simulink model "Buck_DCM_z"  (R2020a)
settings: Solver=FixedStepAuto  StartTime=0.0  StopTime=20  FixedStep=T  RelTol=1e-3
undefined symbols (not defined in the file): C, Iumax, J, Ki_I, Ki_IL, Kp_I, Kp_IL, Kp_Uc, Kp_W, Kphi, L, Lu, rL, Ru, T, Ubat
libraries: powerlib_meascontrol x3
settings Model: Creator=Nguyen Tung  LastModifiedBy=Nguyen Tung

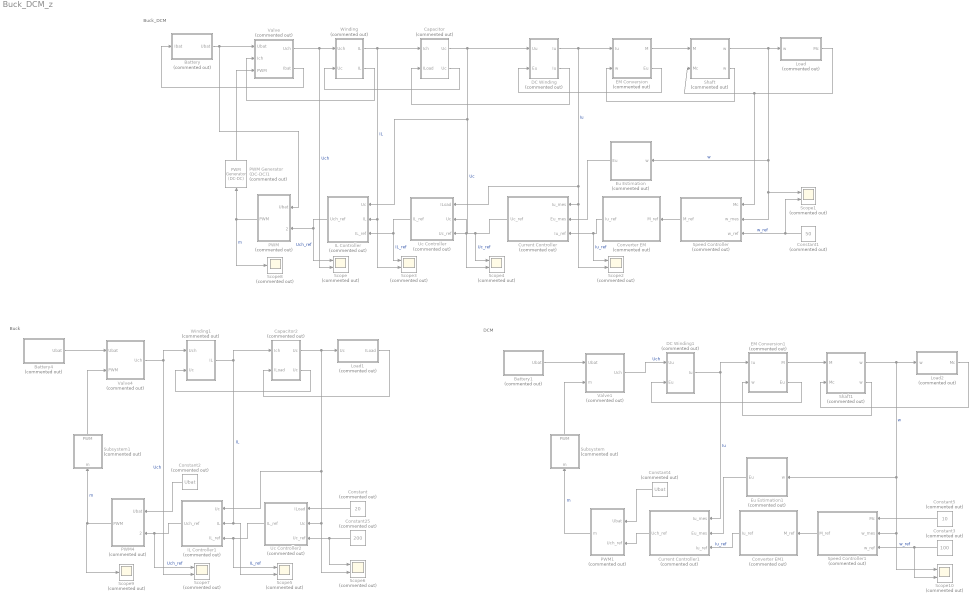
== system Buck_DCM_z ==
  note: DCM
  note: Buck
  note: Buck_DCM
  Battery : Subsystem  Commented=on  AncestorBlock=simulink/REM/SE
      mask Display:
      | plot(0,0,100,100, 1.2*[50,57.68,60.77,63.08,64.97,66.58,68,69.26,70.4, 	71.42,72.36,78.28,80,78.28,72.36,71.42,70.4, 	69.26,68,66.58,64.97,63.08,60.77,57.68,50,42.32, 	39.23,36.92,35.03,33.42,32,30.74,29.6,28.58, 	27.64,21.72,20,21.72,27.64,28.58,29.6,30.74,32, 	33.42,35.03,36.92,39.23,42.32,50]-10, 1.2*[20,21,22,23,24,25,26,27,28,29,30,40,50,60,70,71,72, 	73,74,75,76,77,78,79,80,79,78,77,76,75,74,73,72, 	71,70,60,50,40,30,29,28,27,26,25,24,23,22,21,20]-10)
      | disp('ES')
  Battery1 : Subsystem  Commented=on  AncestorBlock=simulink/REM/SE
      mask Display:
      | plot(0,0,100,100, 1.2*[50,57.68,60.77,63.08,64.97,66.58,68,69.26,70.4, 	71.42,72.36,78.28,80,78.28,72.36,71.42,70.4, 	69.26,68,66.58,64.97,63.08,60.77,57.68,50,42.32, 	39.23,36.92,35.03,33.42,32,30.74,29.6,28.58, 	27.64,21.72,20,21.72,27.64,28.58,29.6,30.74,32, 	33.42,35.03,36.92,39.23,42.32,50]-10, 1.2*[20,21,22,23,24,25,26,27,28,29,30,40,50,60,70,71,72, 	73,74,75,76,77,78,79,80,79,78,77,76,75,74,73,72, 	71,70,60,50,40,30,29,28,27,26,25,24,23,22,21,20]-10)
      | disp('ES')
  Battery4 : Subsystem  Commented=on  AncestorBlock=simulink/REM/SE
      mask Display:
      | plot(0,0,100,100, 1.2*[50,57.68,60.77,63.08,64.97,66.58,68,69.26,70.4, 	71.42,72.36,78.28,80,78.28,72.36,71.42,70.4, 	69.26,68,66.58,64.97,63.08,60.77,57.68,50,42.32, 	39.23,36.92,35.03,33.42,32,30.74,29.6,28.58, 	27.64,21.72,20,21.72,27.64,28.58,29.6,30.74,32, 	33.42,35.03,36.92,39.23,42.32,50]-10, 1.2*[20,21,22,23,24,25,26,27,28,29,30,40,50,60,70,71,72, 	73,74,75,76,77,78,79,80,79,78,77,76,75,74,73,72, 	71,70,60,50,40,30,29,28,27,26,25,24,23,22,21,20]-10)
      | disp('ES')
  Capacitor : Subsystem  Commented=on  AncestorBlock=simulink/REM/EA  mask(CM){}
      mask Display: plot(0,0,100,100,[10,10,90,90,10],[90,10,10,90,90], [10,90],[10,90])
  Capacitor2 : Subsystem  Commented=on  AncestorBlock=simulink/REM/EA  mask(CM){}
      mask Display: plot(0,0,100,100,[10,10,90,90,10],[90,10,10,90,90], [10,90],[10,90])
  Constant : Constant  Commented=on  Value=20
  Constant1 : Constant  Commented=on  Value=50
  Constant2 : Constant  Commented=on  Value=Ubat
  Constant25 : Constant  Commented=on  Value=200  SampleTime=T
  Constant3 : Constant  Commented=on  Value=100
  Constant4 : Constant  Commented=on  Value=Ubat
  Constant5 : Constant  Commented=on  Value=10
  Converter EM : Subsystem  Commented=on  AncestorBlock=simulink/SMC/Inversion EC avec mesure
      mask Display: plot(0,0,100,100,[10,30,90,70,10],[90,10,10,90,90])
  Converter EM1 : Subsystem  Commented=on  AncestorBlock=simulink/SMC/Inversion EC avec mesure
      mask Display: plot(0,0,100,100,[10,30,90,70,10],[90,10,10,90,90])
  Current Controller : Subsystem  Commented=on  AncestorBlock=simulink/SMC/Asservissement Correcteur IP
      mask Display: plot(0,0,100,100, [10,30,90,70,10,90],[90,10,10,90,90,10])
  Current Controller1 : Subsystem  Commented=on  AncestorBlock=simulink/SMC/Asservissement Correcteur IP
      mask Display: plot(0,0,100,100, [10,30,90,70,10,90],[90,10,10,90,90,10])
  DC Winding : Subsystem  Commented=on  AncestorBlock=simulink/REM/EA  mask(CM){}
      mask Display: plot(0,0,100,100,[10,10,90,90,10],[90,10,10,90,90], [10,90],[10,90])
  DC Winding1 : Subsystem  Commented=on  AncestorBlock=simulink/REM/EA  mask(CM){}
      mask Display: plot(0,0,100,100,[10,10,90,90,10],[90,10,10,90,90], [10,90],[10,90])
  EM Conversion : Subsystem  Commented=on  AncestorBlock=simulink/REM/EC EM
      mask Display: plot(0,0,100,100, 1.4*[50,57.68,60.77,63.08,64.97,66.58,68,69.26,70.4, 	71.42,72.36,78.28,80,78.28,72.36,71.42,70.4, 	69.26,68,66.58,64.97,63.08,60.77,57.68,50,42.32, 	39.23,36.92,35.03,33.42,32,30.74,29.6,28.58, 	27.64,21.72,20,21.72,27.64,28.58,29.6,30.74,32, 	33.42,35.03,36.92,39.23,42.32,50]-20, 1.4*[20,21,22,23,24,25,26,27,28,29,30,40,50,60,70,71,72, 	73,74,75,76,77,78,79,80,79,78,77,76,75,74,73,72, 	71,70,60,50,40,30,29,28,27,26,25,24,23,22,21,20]-20)
  EM Conversion1 : Subsystem  Commented=on  AncestorBlock=simulink/REM/EC EM
      mask Display: plot(0,0,100,100, 1.4*[50,57.68,60.77,63.08,64.97,66.58,68,69.26,70.4, 	71.42,72.36,78.28,80,78.28,72.36,71.42,70.4, 	69.26,68,66.58,64.97,63.08,60.77,57.68,50,42.32, 	39.23,36.92,35.03,33.42,32,30.74,29.6,28.58, 	27.64,21.72,20,21.72,27.64,28.58,29.6,30.74,32, 	33.42,35.03,36.92,39.23,42.32,50]-20, 1.4*[20,21,22,23,24,25,26,27,28,29,30,40,50,60,70,71,72, 	73,74,75,76,77,78,79,80,79,78,77,76,75,74,73,72, 	71,70,60,50,40,30,29,28,27,26,25,24,23,22,21,20]-20)
  Eu Estimation : Subsystem  Commented=on  AncestorBlock=simulink/REM/EC EM
      mask Display: plot(0,0,100,100, 1.4*[50,57.68,60.77,63.08,64.97,66.58,68,69.26,70.4, 	71.42,72.36,78.28,80,78.28,72.36,71.42,70.4, 	69.26,68,66.58,64.97,63.08,60.77,57.68,50,42.32, 	39.23,36.92,35.03,33.42,32,30.74,29.6,28.58, 	27.64,21.72,20,21.72,27.64,28.58,29.6,30.74,32, 	33.42,35.03,36.92,39.23,42.32,50]-20, 1.4*[20,21,22,23,24,25,26,27,28,29,30,40,50,60,70,71,72, 	73,74,75,76,77,78,79,80,79,78,77,76,75,74,73,72, 	71,70,60,50,40,30,29,28,27,26,25,24,23,22,21,20]-20)
  Eu Estimation1 : Subsystem  Commented=on  AncestorBlock=simulink/REM/EC EM
      mask Display: plot(0,0,100,100, 1.4*[50,57.68,60.77,63.08,64.97,66.58,68,69.26,70.4, 	71.42,72.36,78.28,80,78.28,72.36,71.42,70.4, 	69.26,68,66.58,64.97,63.08,60.77,57.68,50,42.32, 	39.23,36.92,35.03,33.42,32,30.74,29.6,28.58, 	27.64,21.72,20,21.72,27.64,28.58,29.6,30.74,32, 	33.42,35.03,36.92,39.23,42.32,50]-20, 1.4*[20,21,22,23,24,25,26,27,28,29,30,40,50,60,70,71,72, 	73,74,75,76,77,78,79,80,79,78,77,76,75,74,73,72, 	71,70,60,50,40,30,29,28,27,26,25,24,23,22,21,20]-20)
  IL Controller : Subsystem  Commented=on  AncestorBlock=simulink/SMC/Asservissement Correcteur IP
      mask Display: plot(0,0,100,100, [10,30,90,70,10,90],[90,10,10,90,90,10])
  IL Controller1 : Subsystem  Commented=on  AncestorBlock=simulink/SMC/Asservissement Correcteur IP
      mask Display: plot(0,0,100,100, [10,30,90,70,10,90],[90,10,10,90,90,10])
  Load : Subsystem  Commented=on  AncestorBlock=simulink/REM/SE
      mask Display:
      | plot(0,0,100,100, 1.2*[50,57.68,60.77,63.08,64.97,66.58,68,69.26,70.4, 	71.42,72.36,78.28,80,78.28,72.36,71.42,70.4, 	69.26,68,66.58,64.97,63.08,60.77,57.68,50,42.32, 	39.23,36.92,35.03,33.42,32,30.74,29.6,28.58, 	27.64,21.72,20,21.72,27.64,28.58,29.6,30.74,32, 	33.42,35.03,36.92,39.23,42.32,50]-10, 1.2*[20,21,22,23,24,25,26,27,28,29,30,40,50,60,70,71,72, 	73,74,75,76,77,78,79,80,79,78,77,76,75,74,73,72, 	71,70,60,50,40,30,29,28,27,26,25,24,23,22,21,20]-10)
      | disp('MS')
  Load1 : Subsystem  Commented=on  AncestorBlock=simulink/REM/SE
      mask Display:
      | plot(0,0,100,100, 1.2*[50,57.68,60.77,63.08,64.97,66.58,68,69.26,70.4, 	71.42,72.36,78.28,80,78.28,72.36,71.42,70.4, 	69.26,68,66.58,64.97,63.08,60.77,57.68,50,42.32, 	39.23,36.92,35.03,33.42,32,30.74,29.6,28.58, 	27.64,21.72,20,21.72,27.64,28.58,29.6,30.74,32, 	33.42,35.03,36.92,39.23,42.32,50]-10, 1.2*[20,21,22,23,24,25,26,27,28,29,30,40,50,60,70,71,72, 	73,74,75,76,77,78,79,80,79,78,77,76,75,74,73,72, 	71,70,60,50,40,30,29,28,27,26,25,24,23,22,21,20]-10)
      | disp('MS')
  Load2 : Subsystem  Commented=on  AncestorBlock=simulink/REM/SE
      mask Display:
      | plot(0,0,100,100, 1.2*[50,57.68,60.77,63.08,64.97,66.58,68,69.26,70.4, 	71.42,72.36,78.28,80,78.28,72.36,71.42,70.4, 	69.26,68,66.58,64.97,63.08,60.77,57.68,50,42.32, 	39.23,36.92,35.03,33.42,32,30.74,29.6,28.58, 	27.64,21.72,20,21.72,27.64,28.58,29.6,30.74,32, 	33.42,35.03,36.92,39.23,42.32,50]-10, 1.2*[20,21,22,23,24,25,26,27,28,29,30,40,50,60,70,71,72, 	73,74,75,76,77,78,79,80,79,78,77,76,75,74,73,72, 	71,70,60,50,40,30,29,28,27,26,25,24,23,22,21,20]-10)
      | disp('MS')
  PWM : Subsystem  Commented=on  AncestorBlock=simulink/SMC/Inversion EC avec mesure
      mask Display: plot(0,0,100,100,[10,30,90,70,10],[90,10,10,90,90])
  PWM Generator (DC-DC)1 : powerlib_meascontrol/Pulse & Signal Generators/PWM Generator (DC-DC)  Commented=on  Fsw=1000  Ts=T
  PWM1 : Subsystem  Commented=on  AncestorBlock=simulink/SMC/Inversion EC avec mesure
      mask Display: plot(0,0,100,100,[10,30,90,70,10],[90,10,10,90,90])
  PWM4 : Subsystem  Commented=on  AncestorBlock=simulink/SMC/Inversion EC avec mesure
      mask Display: plot(0,0,100,100,[10,30,90,70,10],[90,10,10,90,90])
  Scope{,1..7,10} (9 alike) : Scope  Commented=on  NumInputPorts=2
  Scope8 : Scope  Commented=on
  Scope9 : Scope  Commented=on
  Shaft : Subsystem  Commented=on  AncestorBlock=simulink/REM/EA  mask(CM){}
      mask Display: plot(0,0,100,100,[10,10,90,90,10],[90,10,10,90,90], [10,90],[10,90])
  Shaft1 : Subsystem  Commented=on  AncestorBlock=simulink/REM/EA  mask(CM){}
      mask Display: plot(0,0,100,100,[10,10,90,90,10],[90,10,10,90,90], [10,90],[10,90])
  Speed Controller : Subsystem  Commented=on  AncestorBlock=simulink/SMC/Asservissement Correcteur IP
      mask Display: plot(0,0,100,100, [10,30,90,70,10,90],[90,10,10,90,90,10])
  Speed Controller1 : Subsystem  Commented=on  AncestorBlock=simulink/SMC/Asservissement Correcteur IP
      mask Display: plot(0,0,100,100, [10,30,90,70,10,90],[90,10,10,90,90,10])
  Subsystem : Subsystem  Commented=on
  Subsystem1 : Subsystem  Commented=on
  Uc Controller : Subsystem  Commented=on  AncestorBlock=simulink/SMC/Asservissement Correcteur IP
      mask Display: plot(0,0,100,100, [10,30,90,70,10,90],[90,10,10,90,90,10])
  Uc Controller2 : Subsystem  Commented=on  AncestorBlock=simulink/SMC/Asservissement Correcteur IP
      mask Display: plot(0,0,100,100, [10,30,90,70,10,90],[90,10,10,90,90,10])
  Valve : Subsystem  Commented=on  AncestorBlock=simulink/REM/EC Elec  mask(Hacheur){}
      mask Display: plot(0,0,100,100,[10,10,90,90,10],[90,10,10,90,90])
  Valve1 : Subsystem  Commented=on  AncestorBlock=simulink/REM/EC Elec  mask(Hacheur){}
      mask Display: plot(0,0,100,100,[10,10,90,90,10],[90,10,10,90,90])
  Valve4 : Subsystem  Commented=on  AncestorBlock=simulink/REM/EC Elec  mask(Hacheur){}
      mask Display: plot(0,0,100,100,[10,10,90,90,10],[90,10,10,90,90])
  Winding : Subsystem  Commented=on  AncestorBlock=simulink/REM/EA  mask(CM){}
      mask Display: plot(0,0,100,100,[10,10,90,90,10],[90,10,10,90,90], [10,90],[10,90])
  Winding1 : Subsystem  Commented=on  AncestorBlock=simulink/REM/EA  mask(CM){}
      mask Display: plot(0,0,100,100,[10,10,90,90,10],[90,10,10,90,90], [10,90],[10,90])
  wires:
  Capacitor/1(Uc) -> DC Winding/1(Uu), IL Controller/1(Uc), Scope4/2, Uc Controller/2(Uc)  "Uc"
  Shaft/1(w) -> Load/1(w), Speed Controller/2(w_mes), Scope1/1, Eu Estimation/1(w)  "w"
  Winding/1(IL) -> Capacitor/1(Ich), Scope3/2, IL Controller/2(IL)  "IL"
  Valve/1(Uch) -> Scope/2, Winding/1(Uch)  "Uch"
  Speed Controller/1(M_ref) -> Converter EM/1(M_ref)
  PWM/1(PWM) -> Scope8/1, PWM Generator (DC-DC)1/1  "m"
  Valve/2(Ibat) -> Battery/1(Ibat)
  Load/1(Mc) -> Speed Controller/1(Mc), Shaft/2(Mc)
  Converter EM/1(Iu_ref) -> Current Controller/3(Iu_ref), Scope2/1  "Iu_ref"
  Uc Controller/1(IL_ref) -> Scope3/1, IL Controller/3(IL_ref)  "IL_ref"
  Shaft/2("w ") -> EM Conversion/2(w)
  EM Conversion/1(M) -> Shaft/1(M)
  EM Conversion/2(Eu) -> DC Winding/2(Eu)
  IL Controller/1(Uch_ref) -> Scope/1, PWM/2(Uch_ref)  "Uch_ref"
  DC Winding/2("Iu ") -> Capacitor/2(ILoad)
  Eu Estimation/1(Eu) -> Current Controller/2(Eu_mes)
  Constant1/1 -> Speed Controller/3(w_ref), Scope1/2  "w_ref"
  DC Winding/1(Iu) -> EM Conversion/1(Iu), Scope2/2, Current Controller/1(Iu_mes), Uc Controller/1(ILoad)  "Iu"
  Battery/1(Ubat) -> Valve/1(Ubat), PWM/1(Ubat)
  Winding/2("IL ") -> Valve/2(Ich)
  Capacitor/2("Uc ") -> Winding/2(Uc)
  Current Controller/1(Uc_ref) -> Scope4/1, Uc Controller/3(Uc_ref)  "Uc_ref"
  PWM4/1(PWM) -> Scope9/1, Subsystem1/1(m)  "m"
  Load1/1(ILoad) -> Capacitor2/2(ILoad)
  Battery4/1(Ubat) -> Valve4/1(Ubat)
  Capacitor2/1(Uc) -> Load1/1(Uc), IL Controller1/1(Uc), Scope6/2, Uc Controller2/2(Uc)
  Winding1/1(IL) -> Capacitor2/1(Ich), Scope5/2, IL Controller1/2(IL)  "IL"
  Valve4/1(Uch) -> Winding1/1(Uch), Scope7/2  "Uch"
  IL Controller1/1(Uch_ref) -> Scope7/1, PWM4/2(Uch_ref)  "Uch_ref"
  Uc Controller2/1(IL_ref) -> Scope5/1, IL Controller1/3(IL_ref)  "IL_ref"
  Capacitor2/2("Uc ") -> Winding1/2(Uc)
  Constant25/1 -> Scope6/1, Uc Controller2/3(Uc_ref)
  PWM Generator (DC-DC)1/1 -> Valve/3(PWM)
  Constant/1 -> Uc Controller2/1(ILoad)
  Constant2/1 -> PWM4/1(Ubat)
  Converter EM1/1(Iu_ref) -> Current Controller1/3(Iu_ref)  "Iu_ref"
  Shaft1/1(w) -> Load2/1(w), Scope10/1, Speed Controller1/2(w_mes), Eu Estimation1/1(w)  "w"
  DC Winding1/1(Iu) -> EM Conversion1/1(Iu), Current Controller1/1(Iu_mes)  "Iu"
  EM Conversion1/2(Eu) -> DC Winding1/2(Eu)
  Eu Estimation1/1(Eu) -> Current Controller1/2(Eu_mes)
  Constant3/1 -> Speed Controller1/3(w_ref), Scope10/2  "w_ref"
  EM Conversion1/1(M) -> Shaft1/1(M)
  Shaft1/2("w ") -> EM Conversion1/2(w)
  Speed Controller1/1(M_ref) -> Converter EM1/1(M_ref)
  Load2/1(Mc) -> Shaft1/2(Mc)
  Battery1/1(Ubat) -> Valve1/1(Ubat)
  Valve1/1(Uch) -> DC Winding1/1(Uu)  "Uch"
  Current Controller1/1(Uch_ref) -> PWM1/2(Uch_ref)
  Constant4/1 -> PWM1/1(Ubat)
  PWM1/1(m) -> Subsystem/1(m)  "m"
  Subsystem/1(PWM) -> Valve1/2(m)
  Subsystem1/1(PWM) -> Valve4/2(PWM)
  Constant5/1 -> Speed Controller1/1(Mc)

== system Buck_DCM_z/Battery ==
  Ibat : Inport
  Constant : Constant  Value=Ubat
  Terminator : Terminator
  Ubat : Outport  InitialOutput=0  VectorParamsAs1DForOutWhenUnconnected=off
  wires:
  Constant/1 -> Ubat/1
  Ibat/1 -> Terminator/1

== system Buck_DCM_z/Battery1 ==
  Constant : Constant  Value=Ubat  SampleTime=T
  Ubat : Outport  InitialOutput=0  VectorParamsAs1DForOutWhenUnconnected=off
  wires:
  Constant/1 -> Ubat/1

== system Buck_DCM_z/Battery4 ==
  Constant : Constant  Value=Ubat  SampleTime=T
  Ubat : Outport  InitialOutput=0  VectorParamsAs1DForOutWhenUnconnected=off
  wires:
  Constant/1 -> Ubat/1

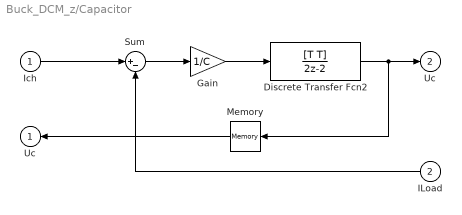
== system Buck_DCM_z/Capacitor ==
  Ich : Inport
  ILoad : Inport  Port=2
  Discrete Transfer Fcn2 : DiscreteTransferFcn  Numerator=[T T]  Denominator=[2 -2]
  Gain : Gain  Gain=1/C
  Memory : Memory
  Sum : Sum  Inputs=|+-
  Uc : Outport  InitialOutput=0  VectorParamsAs1DForOutWhenUnconnected=off
  "Uc " : Outport  Port=2  InitialOutput=0  VectorParamsAs1DForOutWhenUnconnected=off
  wires:
  Ich/1 -> Sum/1
  Sum/1 -> Gain/1
  Gain/1 -> Discrete Transfer Fcn2/1
  Discrete Transfer Fcn2/1 -> "Uc "/1, Memory/1
  ILoad/1 -> Sum/2
  Memory/1 -> Uc/1

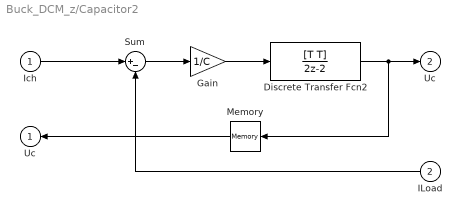
== system Buck_DCM_z/Capacitor2 ==
  Ich : Inport
  ILoad : Inport  Port=2
  Discrete Transfer Fcn2 : DiscreteTransferFcn  Numerator=[T T]  Denominator=[2 -2]
  Gain : Gain  Gain=1/C
  Memory : Memory
  Sum : Sum  Inputs=|+-
  Uc : Outport  InitialOutput=0  VectorParamsAs1DForOutWhenUnconnected=off
  "Uc " : Outport  Port=2  InitialOutput=0  VectorParamsAs1DForOutWhenUnconnected=off
  wires:
  Ich/1 -> Sum/1
  Sum/1 -> Gain/1
  Gain/1 -> Discrete Transfer Fcn2/1
  Discrete Transfer Fcn2/1 -> "Uc "/1, Memory/1
  ILoad/1 -> Sum/2
  Memory/1 -> Uc/1

== system Buck_DCM_z/Converter EM ==
  M_ref : Inport
  Gain : Gain  Gain=1/Kphi
  Saturation : Saturate  Commented=through  UpperLimit=Iumax  LowerLimit=0
  Iu_ref : Outport  InitialOutput=0  VectorParamsAs1DForOutWhenUnconnected=off
  wires:
  M_ref/1 -> Gain/1
  Gain/1 -> Saturation/1
  Saturation/1 -> Iu_ref/1

== system Buck_DCM_z/Converter EM1 ==
  M_ref : Inport
  Gain : Gain  Gain=1/Kphi
  Saturation : Saturate  Commented=through  UpperLimit=Iumax  LowerLimit=0
  Iu_ref : Outport  InitialOutput=0  VectorParamsAs1DForOutWhenUnconnected=off
  wires:
  M_ref/1 -> Gain/1
  Gain/1 -> Saturation/1
  Saturation/1 -> Iu_ref/1

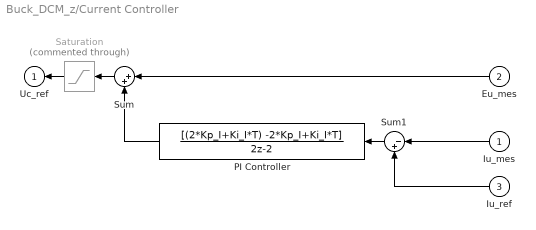
== system Buck_DCM_z/Current Controller ==
  Iu_mes : Inport
  Eu_mes : Inport  Port=2
  Iu_ref : Inport  Port=3
  PI Controller : DiscreteTransferFcn  Numerator=[(2*Kp_I+Ki_I*T) -2*Kp_I+Ki_I*T]  Denominator=[2 -2]
  Saturation : Saturate  Commented=through  UpperLimit=Ubat  LowerLimit=0
  Sum : Sum  Inputs=|++
  Sum1 : Sum  Inputs=|-+
  Uc_ref : Outport  InitialOutput=0  VectorParamsAs1DForOutWhenUnconnected=off
  wires:
  Eu_mes/1 -> Sum/1
  Iu_mes/1 -> Sum1/1
  Sum1/1 -> PI Controller/1
  PI Controller/1 -> Sum/2
  Iu_ref/1 -> Sum1/2
  Sum/1 -> Saturation/1
  Saturation/1 -> Uc_ref/1

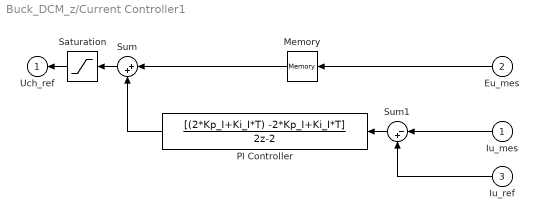
== system Buck_DCM_z/Current Controller1 ==
  Iu_mes : Inport
  Eu_mes : Inport  Port=2
  Iu_ref : Inport  Port=3
  Memory : Memory
  PI Controller : DiscreteTransferFcn  Numerator=[(2*Kp_I+Ki_I*T) -2*Kp_I+Ki_I*T]  Denominator=[2 -2]
  Saturation : Saturate  UpperLimit=Ubat  LowerLimit=0
  Sum : Sum  Inputs=|++
  Sum1 : Sum  Inputs=|-+
  Uch_ref : Outport  InitialOutput=0  VectorParamsAs1DForOutWhenUnconnected=off
  wires:
  Eu_mes/1 -> Memory/1
  Iu_mes/1 -> Sum1/1
  Sum1/1 -> PI Controller/1
  PI Controller/1 -> Sum/2
  Iu_ref/1 -> Sum1/2
  Sum/1 -> Saturation/1
  Saturation/1 -> Uch_ref/1
  Memory/1 -> Sum/1

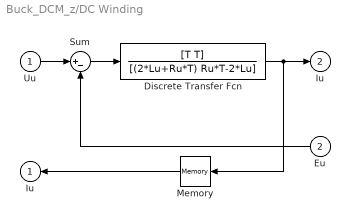
== system Buck_DCM_z/DC Winding ==
  Uu : Inport
  Eu : Inport  Port=2
  Discrete Transfer Fcn : DiscreteTransferFcn  Numerator=[T T]  Denominator=[(2*Lu+Ru*T) Ru*T-2*Lu]
  Memory : Memory
  Sum : Sum  Inputs=|+-
  Iu : Outport  InitialOutput=0  VectorParamsAs1DForOutWhenUnconnected=off
  "Iu " : Outport  Port=2  InitialOutput=0  VectorParamsAs1DForOutWhenUnconnected=off
  wires:
  Uu/1 -> Sum/1
  Sum/1 -> Discrete Transfer Fcn/1
  Discrete Transfer Fcn/1 -> Memory/1, "Iu "/1
  Eu/1 -> Sum/2
  Memory/1 -> Iu/1

== system Buck_DCM_z/DC Winding1 ==
  Uu : Inport
  Eu : Inport  Port=2
  Discrete Transfer Fcn : DiscreteTransferFcn  Numerator=[T T]  Denominator=[(2*Lu+Ru*T) Ru*T-2*Lu]
  Memory : Memory
  Sum : Sum  Inputs=|+-
  Iu : Outport  InitialOutput=0  VectorParamsAs1DForOutWhenUnconnected=off
  wires:
  Uu/1 -> Sum/1
  Sum/1 -> Discrete Transfer Fcn/1
  Discrete Transfer Fcn/1 -> Iu/1
  Eu/1 -> Memory/1
  Memory/1 -> Sum/2

== system Buck_DCM_z/EM Conversion ==
  Iu : Inport
  w : Inport  Port=2
  Gain : Gain  Gain=Kphi
  Gain1 : Gain  Gain=Kphi
  M : Outport  InitialOutput=0  VectorParamsAs1DForOutWhenUnconnected=off
  Eu : Outport  Port=2  InitialOutput=0  VectorParamsAs1DForOutWhenUnconnected=off
  wires:
  Iu/1 -> Gain/1
  Gain/1 -> M/1
  w/1 -> Gain1/1
  Gain1/1 -> Eu/1

== system Buck_DCM_z/EM Conversion1 ==
  Iu : Inport
  w : Inport  Port=2
  Gain : Gain  Gain=Kphi
  Gain1 : Gain  Gain=Kphi
  M : Outport  InitialOutput=0  VectorParamsAs1DForOutWhenUnconnected=off
  Eu : Outport  Port=2  InitialOutput=0  VectorParamsAs1DForOutWhenUnconnected=off
  wires:
  Iu/1 -> Gain/1
  Gain/1 -> M/1
  w/1 -> Gain1/1
  Gain1/1 -> Eu/1

== system Buck_DCM_z/Eu Estimation ==
  w : Inport
  Gain1 : Gain  Gain=Kphi
  Eu : Outport  InitialOutput=0  VectorParamsAs1DForOutWhenUnconnected=off
  wires:
  w/1 -> Gain1/1
  Gain1/1 -> Eu/1

== system Buck_DCM_z/Eu Estimation1 ==
  w : Inport
  Gain1 : Gain  Gain=Kphi
  Eu : Outport  InitialOutput=0  VectorParamsAs1DForOutWhenUnconnected=off
  wires:
  w/1 -> Gain1/1
  Gain1/1 -> Eu/1

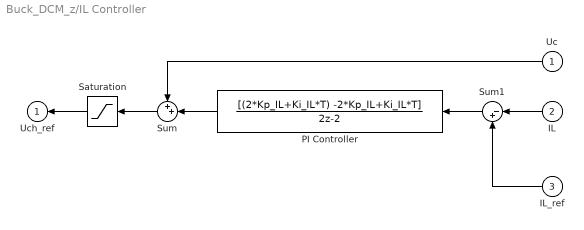
== system Buck_DCM_z/IL Controller ==
  Uc : Inport
  IL : Inport  Port=2
  IL_ref : Inport  Port=3
  PI Controller : DiscreteTransferFcn  Numerator=[(2*Kp_IL+Ki_IL*T) -2*Kp_IL+Ki_IL*T]  Denominator=[2 -2]
  Saturation : Saturate  UpperLimit=Ubat  LowerLimit=0
  Sum : Sum  Inputs=++|
  Sum1 : Sum  Inputs=|-+
  Uch_ref : Outport  InitialOutput=0
  wires:
  Uc/1 -> Sum/1
  IL_ref/1 -> Sum1/2
  IL/1 -> Sum1/1
  Sum/1 -> Saturation/1
  PI Controller/1 -> Sum/2
  Sum1/1 -> PI Controller/1
  Saturation/1 -> Uch_ref/1

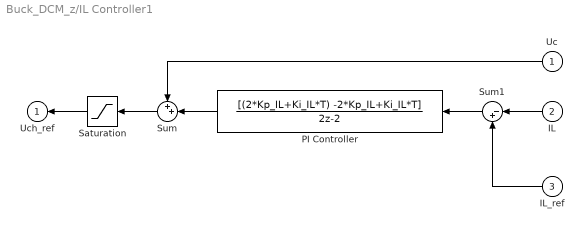
== system Buck_DCM_z/IL Controller1 ==
  Uc : Inport
  IL : Inport  Port=2
  IL_ref : Inport  Port=3
  PI Controller : DiscreteTransferFcn  Numerator=[(2*Kp_IL+Ki_IL*T) -2*Kp_IL+Ki_IL*T]  Denominator=[2 -2]
  Saturation : Saturate  UpperLimit=Ubat  LowerLimit=0
  Sum : Sum  Inputs=++|
  Sum1 : Sum  Inputs=|-+
  Uch_ref : Outport  InitialOutput=0
  wires:
  Uc/1 -> Sum/1
  IL_ref/1 -> Sum1/2
  IL/1 -> Sum1/1
  Sum/1 -> Saturation/1
  Saturation/1 -> Uch_ref/1
  PI Controller/1 -> Sum/2
  Sum1/1 -> PI Controller/1

== system Buck_DCM_z/Load ==
  w : Inport
  Load : Step  Time=5  After=10  SampleTime=T
  Terminator : Terminator
  Mc : Outport  InitialOutput=0  VectorParamsAs1DForOutWhenUnconnected=off
  wires:
  w/1 -> Terminator/1
  Load/1 -> Mc/1

== system Buck_DCM_z/Load1 ==
  Uc : Inport
  Gain : Gain  Gain=1/10
  ILoad : Outport  InitialOutput=0  VectorParamsAs1DForOutWhenUnconnected=off
  wires:
  Uc/1 -> Gain/1
  Gain/1 -> ILoad/1

== system Buck_DCM_z/Load2 ==
  w : Inport
  Load : Step  Time=10  After=10  SampleTime=T
  Terminator : Terminator
  Mc : Outport  InitialOutput=0  VectorParamsAs1DForOutWhenUnconnected=off
  wires:
  w/1 -> Terminator/1
  Load/1 -> Mc/1

== system Buck_DCM_z/PWM ==
  Ubat : Inport
  Uch_ref : Inport  Port=2
  Divide : Product  Inputs=/*
  PWM : Outport
  wires:
  Divide/1 -> PWM/1
  Ubat/1 -> Divide/1
  Uch_ref/1 -> Divide/2

== system Buck_DCM_z/PWM1 ==
  Ubat : Inport
  Uch_ref : Inport  Port=2
  Divide : Product  Inputs=/*
  m : Outport
  wires:
  Ubat/1 -> Divide/1
  Uch_ref/1 -> Divide/2
  Divide/1 -> m/1

== system Buck_DCM_z/PWM4 ==
  Ubat : Inport
  Uch_ref : Inport  Port=2
  Divide : Product  Inputs=/*
  PWM : Outport
  wires:
  Ubat/1 -> Divide/1
  Uch_ref/1 -> Divide/2
  Divide/1 -> PWM/1

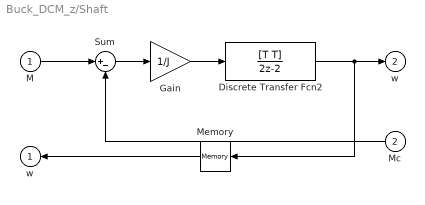
== system Buck_DCM_z/Shaft ==
  M : Inport
  Mc : Inport  Port=2
  Discrete Transfer Fcn2 : DiscreteTransferFcn  Numerator=[T T]  Denominator=[2 -2]
  Gain : Gain  Gain=1/J
  Memory : Memory
  Sum : Sum  Inputs=|+-
  w : Outport  InitialOutput=0  VectorParamsAs1DForOutWhenUnconnected=off
  "w " : Outport  Port=2  InitialOutput=0  VectorParamsAs1DForOutWhenUnconnected=off
  wires:
  M/1 -> Sum/1
  Mc/1 -> Sum/2
  Sum/1 -> Gain/1
  Discrete Transfer Fcn2/1 -> Memory/1, "w "/1
  Gain/1 -> Discrete Transfer Fcn2/1
  Memory/1 -> w/1

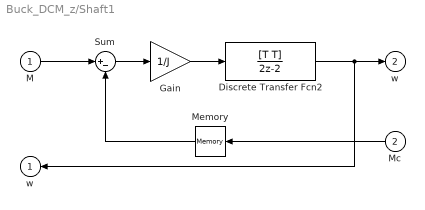
== system Buck_DCM_z/Shaft1 ==
  M : Inport
  Mc : Inport  Port=2
  Discrete Transfer Fcn2 : DiscreteTransferFcn  Numerator=[T T]  Denominator=[2 -2]
  Gain : Gain  Gain=1/J
  Memory : Memory
  Sum : Sum  Inputs=|+-
  w : Outport  InitialOutput=0  VectorParamsAs1DForOutWhenUnconnected=off
  "w " : Outport  Port=2  InitialOutput=0  VectorParamsAs1DForOutWhenUnconnected=off
  wires:
  M/1 -> Sum/1
  Mc/1 -> Memory/1
  Sum/1 -> Gain/1
  Gain/1 -> Discrete Transfer Fcn2/1
  Discrete Transfer Fcn2/1 -> w/1, "w "/1
  Memory/1 -> Sum/2

== system Buck_DCM_z/Speed Controller ==
  Mc : Inport
  w_mes : Inport  Port=2
  w_ref : Inport  Port=3
  P Controller : Gain  Gain=Kp_W
  Sum : Sum  Inputs=|++
  Sum1 : Sum  Inputs=|-+
  M_ref : Outport  InitialOutput=0  VectorParamsAs1DForOutWhenUnconnected=off
  wires:
  Sum/1 -> M_ref/1
  w_ref/1 -> Sum1/2
  Sum1/1 -> P Controller/1
  P Controller/1 -> Sum/2
  Mc/1 -> Sum/1
  w_mes/1 -> Sum1/1

== system Buck_DCM_z/Speed Controller1 ==
  Mc : Inport
  w_mes : Inport  Port=2
  w_ref : Inport  Port=3
  P Controller : Gain  Gain=Kp_W
  Sum : Sum  Inputs=|++
  Sum1 : Sum  Inputs=|-+
  M_ref : Outport  InitialOutput=0  VectorParamsAs1DForOutWhenUnconnected=off
  wires:
  Sum/1 -> M_ref/1
  w_ref/1 -> Sum1/2
  Sum1/1 -> P Controller/1
  P Controller/1 -> Sum/2
  Mc/1 -> Sum/1
  w_mes/1 -> Sum1/1

== system Buck_DCM_z/Subsystem ==
  m : Inport
  Gain : Gain  Gain=255
  PWM Generator (DC-DC) : powerlib_meascontrol/Pulse & Signal Generators/PWM Generator (DC-DC)  Fsw=1000  Ts=T
  PWM : Outport
  wires:
  Gain/1 -> PWM Generator (DC-DC)/1
  PWM Generator (DC-DC)/1 -> PWM/1
  m/1 -> Gain/1

== system Buck_DCM_z/Subsystem1 ==
  m : Inport
  Gain : Gain  Gain=255
  PWM Generator (DC-DC) : powerlib_meascontrol/Pulse & Signal Generators/PWM Generator (DC-DC)  Fsw=1000  Ts=T
  PWM : Outport
  wires:
  m/1 -> Gain/1
  PWM Generator (DC-DC)/1 -> PWM/1
  Gain/1 -> PWM Generator (DC-DC)/1

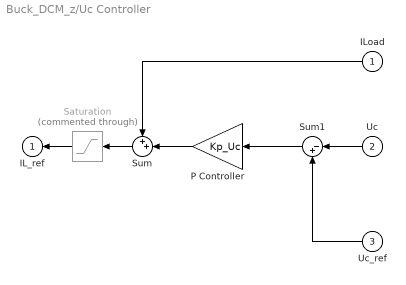
== system Buck_DCM_z/Uc Controller ==
  ILoad : Inport
  Uc : Inport  Port=2
  Uc_ref : Inport  Port=3
  P Controller : Gain  Gain=Kp_Uc
  Saturation : Saturate  Commented=through  UpperLimit=Iumax  LowerLimit=0
  Sum : Sum  Inputs=++|
  Sum1 : Sum  Inputs=|-+
  IL_ref : Outport  InitialOutput=0
  wires:
  Uc/1 -> Sum1/1
  Uc_ref/1 -> Sum1/2
  Sum1/1 -> P Controller/1
  P Controller/1 -> Sum/2
  ILoad/1 -> Sum/1
  Sum/1 -> Saturation/1
  Saturation/1 -> IL_ref/1

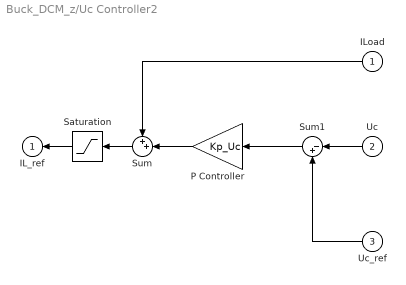
== system Buck_DCM_z/Uc Controller2 ==
  ILoad : Inport
  Uc : Inport  Port=2
  Uc_ref : Inport  Port=3
  P Controller : Gain  Gain=Kp_Uc
  Saturation : Saturate  UpperLimit=60  LowerLimit=0
  Sum : Sum  Inputs=++|
  Sum1 : Sum  Inputs=|-+
  IL_ref : Outport  InitialOutput=0
  wires:
  Uc/1 -> Sum1/1
  Uc_ref/1 -> Sum1/2
  Sum1/1 -> P Controller/1
  P Controller/1 -> Sum/2
  ILoad/1 -> Sum/1
  Sum/1 -> Saturation/1
  Saturation/1 -> IL_ref/1

== system Buck_DCM_z/Valve ==
  Ubat : Inport
  Ich : Inport  Port=2
  PWM : Inport  Port=3
  Product : Product
  Product1 : Product
  Uch : Outport  InitialOutput=0  VectorParamsAs1DForOutWhenUnconnected=off
  Ibat : Outport  Port=2  InitialOutput=0  VectorParamsAs1DForOutWhenUnconnected=off
  wires:
  Product/1 -> Uch/1
  Ubat/1 -> Product/1
  PWM/1 -> Product1/2, Product/2
  Ich/1 -> Product1/1
  Product1/1 -> Ibat/1

== system Buck_DCM_z/Valve1 ==
  Ubat : Inport
  m : Inport  Port=2
  Product : Product
  Uch : Outport  InitialOutput=0  VectorParamsAs1DForOutWhenUnconnected=off
  wires:
  Product/1 -> Uch/1
  Ubat/1 -> Product/1
  m/1 -> Product/2

== system Buck_DCM_z/Valve4 ==
  Ubat : Inport
  PWM : Inport  Port=2
  Product : Product
  Uch : Outport  InitialOutput=0  VectorParamsAs1DForOutWhenUnconnected=off
  wires:
  Product/1 -> Uch/1
  Ubat/1 -> Product/1
  PWM/1 -> Product/2

== system Buck_DCM_z/Winding ==
  Uch : Inport
  Uc : Inport  Port=2
  Discrete Transfer Fcn : DiscreteTransferFcn  Numerator=[T T]  Denominator=[(2*L+rL*T) rL*T-2*L]
  Memory : Memory
  Sum : Sum  Inputs=|+-
  IL : Outport  InitialOutput=0  VectorParamsAs1DForOutWhenUnconnected=off
  "IL " : Outport  Port=2  InitialOutput=0  VectorParamsAs1DForOutWhenUnconnected=off
  wires:
  Uch/1 -> Sum/1
  Discrete Transfer Fcn/1 -> "IL "/1, Memory/1
  Sum/1 -> Discrete Transfer Fcn/1
  Uc/1 -> Sum/2
  Memory/1 -> IL/1

== system Buck_DCM_z/Winding1 ==
  Uch : Inport
  Uc : Inport  Port=2
  Discrete Transfer Fcn : DiscreteTransferFcn  Numerator=[T T]  Denominator=[(2*L+rL*T) rL*T-2*L]
  Sum : Sum  Inputs=|+-
  IL : Outport  InitialOutput=0  VectorParamsAs1DForOutWhenUnconnected=off
  wires:
  Uch/1 -> Sum/1
  Discrete Transfer Fcn/1 -> IL/1
  Sum/1 -> Discrete Transfer Fcn/1
  Uc/1 -> Sum/2
